simulink model "TwentyfourPulseDiodeRectifier"  (R2024b)
settings: Solver=FixedStepDiscrete  StartTime=0.0  StopTime=0.05  FixedStep=5e-5  MaxStep=1e-4  RelTol=1e-3  EnableMultiTasking=on
libraries: fl_lib x16, ee_lib x7, nesl_utility x4
CloseFcn:
  | try,close(h1_TwentyfourPulseDiodeRectifier),end
  | clear h1_TwentyfourPulseDiodeRectifier
  | clear tout simlog_TwentyfourPulseDiodeRectifier
settings Model: Creator=The MathWorks, Inc.  LastModifiedBy=HP
settings SolverCC: MaxConsecutiveZCs=10000  AlgebraicLoopSolver=TrustRegion
settings DataIOCC: LimitDataPoints=on  SaveFormat=Array  ReturnWorkspaceOutputs=off  SignalLoggingName=logsout_TwentyfourPulseDiodeRectifier
settings OptimizationCC: ExpressionDepthLimit=2147483647  LifeSpan=inf
settings DebuggingCC: UnderspecifiedInitializationDetection=Classic  MergeDetectMultiDrivingBlocksExec=none  SolverPrmCheckMsg=warning  MultiTaskDSMMsg=warning  MultiTaskCondExecSysMsg=none  FcnCallInpInsideContextMsg=warning  UnconnectedInputMsg=warning  UnconnectedOutputMsg=warning  UnconnectedLineMsg=warning  StateNameClashWarn=warning  SFUnexpectedBacktrackingDiag=warning  SFNoUnconditionalDefaultTransitionDiag=warning  SFExecutionAtInitializationDiag=none  ArithmeticOperatorsInVariantConditions=warning
settings HardwareCC: ProdBitPerPointer=32  ProdBitPerSizeT=32  ProdBitPerPtrDiffT=32  ProdLargestAtomicFloat=None  ProdIntDivRoundTo=Undefined  ProdEndianess=Unspecified  ProdWordSize=32  ProdHWDeviceType=32-bit Generic
settings ModelReferenceCC: EnableRefExpFcnMdlSchedulingChecks=on  PropagateSignalLabelsOutOfModel=off
settings SFSimCC: SimUseLocalCustomCode=off  CustomCodeUndefinedFunction=UseInterfaceOnly
settings RTWCC: RTWUseLocalCustomCode=off  GPUComputeCapability=3.5
settings CodeAppCC: StateflowObjectComments=on
settings GRTTargetCC: TargetLangStandard=C89/C90 (ANSI)  CombineOutputUpdateFcns=off  GRTInterface=on
settings ConfigComp: CovMetricSettings=dw  CovSaveCumulativeToWorkspaceVar=on  CovSaveSingleToWorkspaceVar=on  CovExternalEMLEnable=off  CovSFcnEnable=off
settings SimscapeCC: SimscapeNormalizeSystem=off  SimscapeNominalValues="[{\"value\":\"10\",\"unit\":\"V\"},{\"value\":\"1\",\"unit\":\"A\"},{\"value\":\"10\",\"unit\":\"N*m\"},{\"value\":\"10\",\"unit\":\"bar\"},{\"value\":\"100\",\"unit\":\"kJ/kg\"},{\"value\":\"1\",\"unit\":\"kW\"},{\"value\":\"300\",\"unit\":\"K\"},{\"value\":\"100\",\"unit\":\"cm^3/s\"},{\"value\":\"1\",\"unit\":\"kN\"},{\"value\":\"1\",\"unit\":\"g/cm^3\"},{\"value\":\"1\",\"unit\":\"l\"},{\"value\":\"1\",\"unit\":\"cm^2\"},{\"value\":\"60\",\"unit\":\"Hz\"}]"  SimscapeLogType=all  SimscapeLogSimulationStatistics=on  SimscapeLogName=simlog_TwentyfourPulseDiodeRectifier  SimscapeLogDataHistory=10000

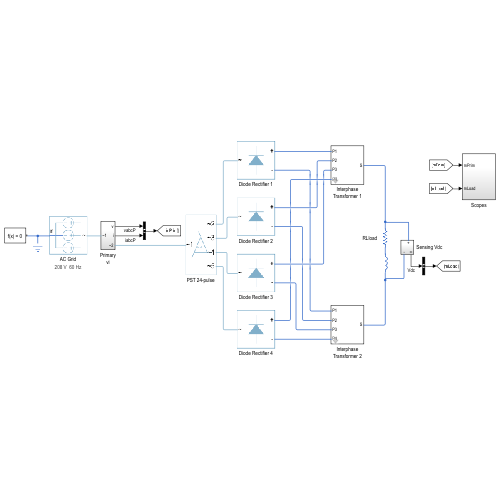
[thumbnail: Simulink's stored preview of the top-level diagram]
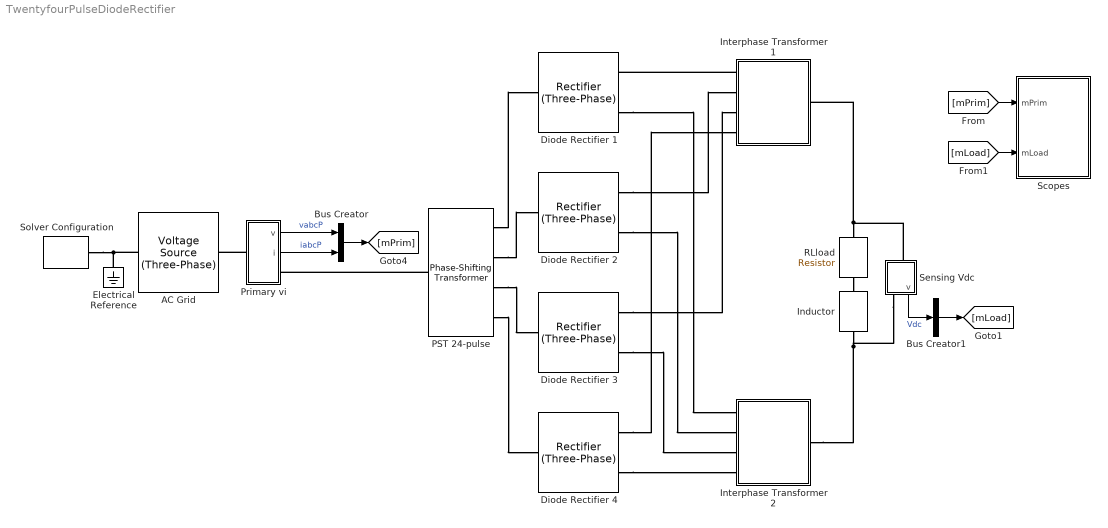
== system TwentyfourPulseDiodeRectifier ==
  AC Grid : ee_lib/Sources/Voltage Source (Three-Phase)  vline_rms=480*sqrt(2)/sqrt(3) V  shift=0 deg  freq=60 Hz  impedance_option=1  SShortCircuit=1e6 A*V  XR=15  R=0.01 Ohm  L=3.97e-4 H  harmonic_option=0  harmonic_orders=[5.0, 7.0, 11.0, 13.0]  harmonic_ratios=[0.1, 0.1, 0.1, 0.1]  G_parasitic=0 1/Ohm  I_specify=off  I_priority=None  I=[0, 0, 0] A  I_nominal_specify=off  I_nominal_value=1  I_nominal_unit=A
      settings: AttributesFormatString="208 V  60 Hz"
  Bus Creator : BusCreator  Inputs=2
  Bus Creator1 : BusCreator  Inputs=1
  Diode Rectifier {1..4} (4 alike) : ee_lib/Semiconductors & Converters/Converters/Rectifier (Three-Phase)  port_option=ee.enum.threePhasePort.composite  Vf=0.8 V  Ron=0.001 Ohm  Goff=1e-5 1/Ohm  model_dynamics=ee.enum.converters.diode.nodynamics  C=50 nF  iRM=-235 A  iF=300 A  idot=-50 A/us  trr_param=1  trr_factor=3  trr=15 us  Qrr=1.5e+3 s*uA
      settings: InternalSimscapePortConfiguration="{\"Bottom\":[],\"Left\":[{\"id\":\"N\",\"label\":\"~\",\"type\":\"foundation.electrical.three_phase\"}],\"Right\":[{\"id\":\"p\",\"label\":\"+\",\"type\":\"foundation.electrical.electrical\"},{\"id\":\"n\",\"label\":\"-\",\"type\":\"foundation.electrical.electrical\"}],\"Top\":[]}"
  Electrical Reference : fl_lib/Electrical/Electrical Elements/Electrical Reference
  Inductor : fl_lib/Electrical/Electrical Elements/Inductor  l=4.24 mH  r=0 Ohm  g=0 1/Ohm  i_specify=off  i_priority=None  i=0 A  i_nominal_specify=off  i_nominal_value=1  i_nominal_unit=A  v_specify=off  v_priority=None  v=0 V  v_nominal_specify=off  v_nominal_value=1  v_nominal_unit=V  i_L_specify=off  i_L_priority=High  i_L=0 A  i_L_nominal_specify=off  i_L_nominal_value=1  i_L_nominal_unit=A
  Interphase Transformer 1 : Subsystem  mask{L=40e-3}
      mask prompts: L "Interphase transformer inductance (H):"
  Interphase Transformer 2 : Subsystem  mask{L=40e-3}
      mask prompts: L "Interphase transformer inductance (H):"
  PST 24-pulse : ee_lib/Passive/Transformers/Phase-Shifting Transformer  pulseNumber=ee.enum.transformer_pulse.twentyfour  SRated=50000 A*V  FRated=60 Hz  VRated=120*sqrt(3) V  pu_Rw1=1e-3  pu_Xl1=1e-3  pu_Rw2=1e-3  pu_Xl2=1e-3  pu_Rm=500  pu_Xm=500  ip_specify=off  ip_priority=None  ip=[0, 0, 0] A  ip_nominal_specify=off  ip_nominal_value=1  ip_nominal_unit=A  is1_specify=off  is1_priority=None  is1=[0, 0, 0] A  is1_nominal_specify=off  is1_nominal_value=1  is1_nominal_unit=A  is2_specify=off  is2_priority=None  is2=[0, 0, 0] A  is2_nominal_specify=off  is2_nominal_value=1  is2_nominal_unit=A  is3_specify=off  is3_priority=None  is3=[0, 0, 0] A  is3_nominal_specify=off  is3_nominal_value=1  is3_nominal_unit=A  is4_specify=off  is4_priority=None  is4=[0, 0, 0] A  is4_nominal_specify=off  is4_nominal_value=1  is4_nominal_unit=A  is5_specify=off  is5_priority=None  is5=[0, 0, 0] A  is5_nominal_specify=off  is5_nominal_value=1  is5_nominal_unit=A  is6_specify=off  is6_priority=None  is6=[0, 0, 0] A  is6_nominal_specify=off  is6_nominal_value=1  is6_nominal_unit=A  is7_specify=off  is7_priority=None  is7=[0, 0, 0] A  is7_nominal_specify=off  is7_nominal_value=1  is7_nominal_unit=A  is8_specify=off  is8_priority=None  is8=[0, 0, 0] A  is8_nominal_specify=off  is8_nominal_value=1  is8_nominal_unit=A  power_dissipated_specify=off  power_dissipated_priority=None  power_dissipated=0 W  power_dissipated_nominal_specify=off  power_dissipated_nominal_value=1  power_dissipated_nominal_unit=W
      settings: InternalSimscapePortConfiguration="{\"Bottom\":[],\"Left\":[{\"id\":\"Np\",\"label\":\"~1\",\"type\":\"foundation.electrical.three_phase\"}],\"Right\":[{\"id\":\"Ns1\",\"label\":\"~2\",\"type\":\"foundation.electrical.three_phase\"},{\"id\":\"Ns2\",\"label\":\"~3\",\"type\":\"foundation.electrical.three_phase\"},{\"id\":\"Ns3\",\"label\":\"~4\",\"type\":\"foundation.electrical.three_phase\"},{\"id\":\"Ns4\",\"label\":\"~5\",\"type\":\"foundation.electrical.three_phase\"}],\"Top\":[]}"
  Primary vi : Subsystem
  RLload : fl_lib/Electrical/Electrical Elements/Resistor  R=2.13 Ohm  i_specify=off  i_priority=High  i=0 A  i_nominal_specify=off  i_nominal_value=1  i_nominal_unit=A  v_specify=off  v_priority=High  v=0 V  v_nominal_specify=off  v_nominal_value=1  v_nominal_unit=V
  Scopes : Subsystem
  Sensing Vdc : Subsystem
      settings: PortSchema="{\"entries\":[{\"content\":{\"sides\":[{\"content\":{\"connectorIds\":[\"LConn1\"]},\"type\":\"ConnectorPlacement.EquallySpacedRectSide\",\"uuid\":\"dd3f0977-3918-40de-94c7-7fbcfbb383a4\"},{\"content\":{\"connectorIds\":[\"RConn1\",\"Out1\"],\"side\":\"RIGHT\"},\"type\":\"ConnectorPlacement.EquallySpacedRectSide\",\"uuid\":\"79db1e6e-d344-4305-b9b8-19f2d8f91918\"},{\"content\":{\"side\":\"TOP\"},\"type\":\"ConnectorPlacement.EquallySpacedRectSide\",\"uuid\":\"ccefdf9b-581f-48d4-aac0-99076ef6e558\"}]},\"type\":\"ConnectorPlacement.EquallySpacedConnector\",\"uuid\":\"19bfc8ea-afa1-4dca-b458-f3c92feb06cb\"}],\"packageUris\":[\"http://schema.mathworks.com/mf0/Connector/R2020b\"],\"version\":\"1.0\"}"
  Solver Configuration : nesl_utility/Solver Configuration  PhysicalDomain=network_engine_domain  SubClassName=solver  LeftPortType=input  RightPortType=generic  Tones=[]  Harmonics=[]  SimulateNoise=off  Profile=off  UseLocalSampling=off  EnableSwitchedLinearOptims=on  FrequencyDomain=off  UseCCode=off  RelTol=0.001  AbsTol=1e-06  MinStep=1e-09  ToWorkspace=off  RevertToSquareIcSolve=off  NumHomotopyIterations=100  PhasorMode=off  PhasorModeNumHarmonics=1  ConsistencySolver=NEWTON_FTOL  IndexReductionMethod=DerivativeReplacement  DoDC=off  ResidualTolerance=1e-09  ConsistencyTolSource=GLOBAL  ConsistencyAbsTol=0.001  ConsistencyRelTol=0.001  ConsistencyTolFactor=0.001  UseLocalSolver=on  LocalSolverChoice=NE_BACKWARD_EULER_ADVANCER  ResolveIndetEquations=on  FunctionEvalNumThread=1  LocalSolverSampleTime=5e-5  DoFixedCost=on  MaxNonlinIter=3  MaxModeIter=2  ComputeImpulses=off  ImpulseIterations=2  LinearAlgebra=auto  LinearAlgebraNumThread=0  EquationFormulation=NE_TIME_EF  DelaysMemoryBudget=1024  AutomaticFiltering=on  FilteringTimeConstant=0.001  PartitionStorageMethod=AS_NEEDED  PartitionMemoryBudget=1024  PartitionMethod=ROBUST  MultibodyUseLocalSolver=off  MultibodyLocalSolverChoice=ODE1  MultibodyLocalSolverSampleTime=0.001
  wires:
  Bus Creator/1 -> [mPrim]
  Primary vi/1(v) -> Bus Creator/1  "vabcP"
  Primary vi/2(i) -> Bus Creator/2  "iabcP"
  Sensing Vdc/1(v) -> Bus Creator1/1  "Vdc"
  Bus Creator1/1 -> [mLoad]
  [mPrim] -> Scopes/1(mPrim)
  [mLoad] -> Scopes/2(mLoad)
  connections:
  Interphase Transformer 2/RConn1 -- Sensing Vdc/RConn1 -- Inductor/RConn1
  Solver Configuration/RConn1 -- Electrical Reference/LConn1 -- AC Grid/LConn1
  PST 24-pulse/RConn2 -- Diode Rectifier 2/LConn1
  PST 24-pulse/RConn1 -- Diode Rectifier 1/LConn1
  Primary vi/LConn1 -- AC Grid/RConn1
  PST 24-pulse/RConn3 -- Diode Rectifier 3/LConn1
  PST 24-pulse/LConn1 -- Primary vi/RConn1
  Sensing Vdc/LConn1 -- Interphase Transformer 1/RConn1 -- RLload/LConn1
  PST 24-pulse/RConn4 -- Diode Rectifier 4/LConn1
  Interphase Transformer 1/LConn1 -- Diode Rectifier 1/RConn1
  Diode Rectifier 2/RConn1 -- Interphase Transformer 1/LConn2
  Diode Rectifier 3/RConn1 -- Interphase Transformer 1/LConn3
  Diode Rectifier 4/RConn1 -- Interphase Transformer 1/LConn4
  Diode Rectifier 1/RConn2 -- Interphase Transformer 2/LConn1
  Diode Rectifier 2/RConn2 -- Interphase Transformer 2/LConn2
  Diode Rectifier 3/RConn2 -- Interphase Transformer 2/LConn3
  Diode Rectifier 4/RConn2 -- Interphase Transformer 2/LConn4
  RLload/RConn1 -- Inductor/LConn1

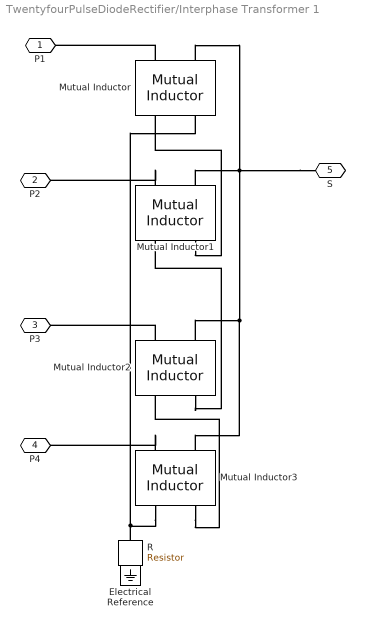
== system TwentyfourPulseDiodeRectifier/Interphase Transformer 1 ==
  Electrical Reference : fl_lib/Electrical/Electrical Elements/Electrical Reference
  Mutual Inductor{,1..3} (4 alike) : fl_lib/Electrical/Electrical Elements/Mutual Inductor  L1=L H  L2=L H  k=0.99999  i1_specify=off  i1_priority=None  i1=0 A  i1_nominal_specify=off  i1_nominal_value=1  i1_nominal_unit=A  i2_specify=off  i2_priority=None  i2=0 A  i2_nominal_specify=off  i2_nominal_value=1  i2_nominal_unit=A  v1_specify=off  v1_priority=None  v1=0 V  v1_nominal_specify=off  v1_nominal_value=1  v1_nominal_unit=V  v2_specify=off  v2_priority=None  v2=0 V  v2_nominal_specify=off  v2_nominal_value=1  v2_nominal_unit=V
      settings: InternalSimscapePortConfiguration="{\"Bottom\":[],\"Left\":[{\"id\":\"p1\",\"label\":\"1+\",\"type\":\"foundation.electrical.electrical\"},{\"id\":\"n1\",\"label\":\"1-\",\"type\":\"foundation.electrical.electrical\"}],\"Right\":[{\"id\":\"p2\",\"label\":\"2+\",\"type\":\"foundation.electrical.electrical\"},{\"id\":\"n2\",\"label\":\"2-\",\"type\":\"foundation.electrical.electrical\"}],\"Top\":[]}"
  R : fl_lib/Electrical/Electrical Elements/Resistor  R=1e9 Ohm  i_specify=off  i_priority=None  i=0 A  i_nominal_specify=off  i_nominal_value=1  i_nominal_unit=A  v_specify=off  v_priority=None  v=0 V  v_nominal_specify=off  v_nominal_value=1  v_nominal_unit=V
  P1 : PMIOPort  Side=Left
  P2 : PMIOPort  Port=2  Side=Left
  P3 : PMIOPort  Port=3  Side=Left
  P4 : PMIOPort  Port=4  Side=Left
  S : PMIOPort  Port=5  Side=Right
  connections:
  Mutual Inductor/RConn2 -- Mutual Inductor3/RConn1 -- R/LConn1
  Mutual Inductor3/RConn2 -- Mutual Inductor2/RConn1
  Mutual Inductor3/LConn1 -- P4/RConn1
  Mutual Inductor2/RConn2 -- Mutual Inductor1/RConn1
  Mutual Inductor1/LConn1 -- P2/RConn1
  Mutual Inductor1/RConn2 -- Mutual Inductor/RConn1
  Mutual Inductor2/LConn1 -- P3/RConn1
  S/RConn1 -- Mutual Inductor2/LConn2 -- Mutual Inductor3/LConn2 -- Mutual Inductor1/LConn2 -- Mutual Inductor/LConn2
  Mutual Inductor/LConn1 -- P1/RConn1
  Electrical Reference/LConn1 -- R/RConn1

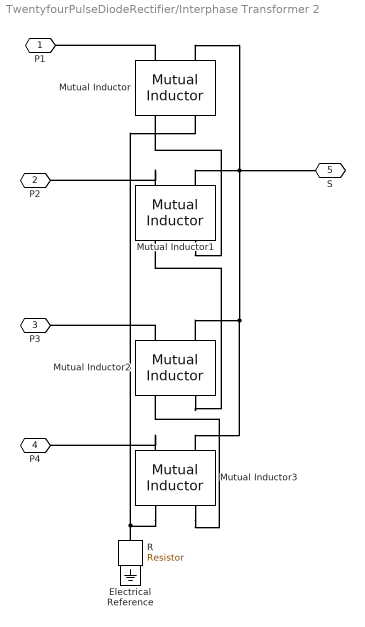
== system TwentyfourPulseDiodeRectifier/Interphase Transformer 2 ==
  Electrical Reference : fl_lib/Electrical/Electrical Elements/Electrical Reference
  Mutual Inductor{,1..3} (4 alike) : fl_lib/Electrical/Electrical Elements/Mutual Inductor  L1=L H  L2=L H  k=0.99999  i1_specify=off  i1_priority=None  i1=0 A  i1_nominal_specify=off  i1_nominal_value=1  i1_nominal_unit=A  i2_specify=off  i2_priority=None  i2=0 A  i2_nominal_specify=off  i2_nominal_value=1  i2_nominal_unit=A  v1_specify=off  v1_priority=None  v1=0 V  v1_nominal_specify=off  v1_nominal_value=1  v1_nominal_unit=V  v2_specify=off  v2_priority=None  v2=0 V  v2_nominal_specify=off  v2_nominal_value=1  v2_nominal_unit=V
      settings: InternalSimscapePortConfiguration="{\"Bottom\":[],\"Left\":[{\"id\":\"p1\",\"label\":\"1+\",\"type\":\"foundation.electrical.electrical\"},{\"id\":\"n1\",\"label\":\"1-\",\"type\":\"foundation.electrical.electrical\"}],\"Right\":[{\"id\":\"p2\",\"label\":\"2+\",\"type\":\"foundation.electrical.electrical\"},{\"id\":\"n2\",\"label\":\"2-\",\"type\":\"foundation.electrical.electrical\"}],\"Top\":[]}"
  R : fl_lib/Electrical/Electrical Elements/Resistor  R=1e9 Ohm  i_specify=off  i_priority=None  i=0 A  i_nominal_specify=off  i_nominal_value=1  i_nominal_unit=A  v_specify=off  v_priority=None  v=0 V  v_nominal_specify=off  v_nominal_value=1  v_nominal_unit=V
  P1 : PMIOPort  Side=Left
  P2 : PMIOPort  Port=2  Side=Left
  P3 : PMIOPort  Port=3  Side=Left
  P4 : PMIOPort  Port=4  Side=Left
  S : PMIOPort  Port=5  Side=Right
  connections:
  Electrical Reference/LConn1 -- R/RConn1
  Mutual Inductor/LConn1 -- P1/RConn1
  Mutual Inductor/LConn2 -- Mutual Inductor1/LConn2 -- Mutual Inductor3/LConn2 -- Mutual Inductor2/LConn2 -- S/RConn1
  Mutual Inductor2/LConn1 -- P3/RConn1
  Mutual Inductor1/RConn2 -- Mutual Inductor/RConn1
  Mutual Inductor1/LConn1 -- P2/RConn1
  Mutual Inductor2/RConn2 -- Mutual Inductor1/RConn1
  Mutual Inductor3/LConn1 -- P4/RConn1
  Mutual Inductor3/RConn2 -- Mutual Inductor2/RConn1
  R/LConn1 -- Mutual Inductor3/RConn1 -- Mutual Inductor/RConn2

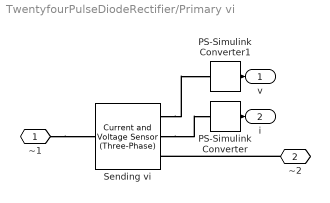
== system TwentyfourPulseDiodeRectifier/Primary vi ==
  PS-Simulink Converter : nesl_utility/PS-Simulink Converter  PhysicalDomain=network_engine_domain  SubClassName=ps_output  LeftPortType=input  RightPortType=output  PseudoPeriodic=off  Frequencies=[]  VectorFormat=1-D array  Unit=A  AffineConversion=off
  PS-Simulink Converter1 : nesl_utility/PS-Simulink Converter  PhysicalDomain=network_engine_domain  SubClassName=ps_output  LeftPortType=input  RightPortType=output  PseudoPeriodic=off  Frequencies=[]  VectorFormat=1-D array  Unit=V  AffineConversion=off
  Sending vi : ee_lib/Sensors & Transducers/Current and Voltage Sensor (Three-Phase)  vMeasurementType=ee.enum.vmeasurement.lg  outputUnit=ee.enum.unit.si  SRated=100e6 A*V  VRated=24e3 V  I_specify=off  I_priority=None  I=[0, 0, 0] A  I_nominal_specify=off  I_nominal_value=1  I_nominal_unit=A  V_specify=off  V_priority=None  V=[0, 0, 0] V  V_nominal_specify=off  V_nominal_value=1  V_nominal_unit=V
      settings: InternalSimscapePortConfiguration="{\"Bottom\":[],\"Left\":[{\"id\":\"N1\",\"label\":\"~1\",\"type\":\"foundation.electrical.three_phase\"}],\"Right\":[{\"id\":\"V_output\",\"label\":\"V\",\"type\":\"output\"},{\"id\":\"I_output\",\"label\":\"I\",\"type\":\"output\"},{\"id\":\"N2\",\"label\":\"~2\",\"type\":\"foundation.electrical.three_phase\"}],\"Top\":[]}"
  ~1 : PMIOPort  Side=Left
  ~2 : PMIOPort  Port=2  Side=Right
  v : Outport
  i : Outport  Port=2
  wires:
  PS-Simulink Converter1/1 -> v/1
  PS-Simulink Converter/1 -> i/1
  connections:
  ~1/RConn1 -- Sending vi/LConn1
  ~2/RConn1 -- Sending vi/RConn3
  Sending vi/RConn1 -- PS-Simulink Converter1/LConn1
  Sending vi/RConn2 -- PS-Simulink Converter/LConn1

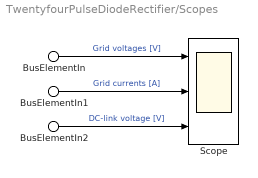
== system TwentyfourPulseDiodeRectifier/Scopes ==
  BusElementIn : Inport  PortName=mPrim  Element=vabcP
  BusElementIn1 : Inport  PortName=mPrim  Element=iabcP
  BusElementIn2 : Inport  Port=2  PortName=mLoad  Element=Vdc
  Scope : Scope  NumInputPorts=3
  wires:
  BusElementIn/1 -> Scope/1  "Grid voltages [V]"
  BusElementIn1/1 -> Scope/2  "Grid currents [A]"
  BusElementIn2/1 -> Scope/3  "DC-link voltage [V]"

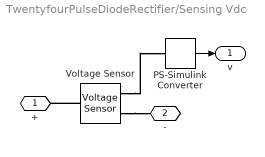
== system TwentyfourPulseDiodeRectifier/Sensing Vdc ==
  PS-Simulink Converter : nesl_utility/PS-Simulink Converter  PhysicalDomain=network_engine_domain  SubClassName=ps_output  LeftPortType=input  RightPortType=output  PseudoPeriodic=off  Frequencies=[]  VectorFormat=1-D array  Unit=V  AffineConversion=off
  Voltage Sensor : fl_lib/Electrical/Electrical Sensors/Voltage Sensor
  + : PMIOPort  Side=Left
  - : PMIOPort  Port=2  Side=Right
  v : Outport
  wires:
  PS-Simulink Converter/1 -> v/1
  connections:
  Voltage Sensor/RConn1 -- PS-Simulink Converter/LConn1
  Voltage Sensor/LConn1 -- +/RConn1
  Voltage Sensor/RConn2 -- -/RConn1
